simulink model "L3_T2_cascade_position"  (R2026a)
settings: Solver=ode23tb  StartTime=0  StopTime=4  MaxStep=0.001
settings Model: Creator=m  LastModifiedBy=m

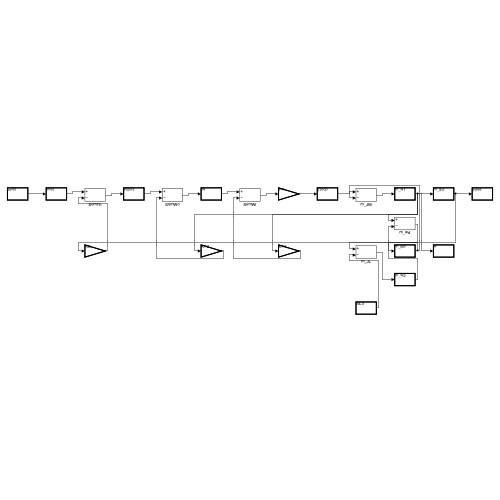
[thumbnail: Simulink's stored preview of the top-level diagram]
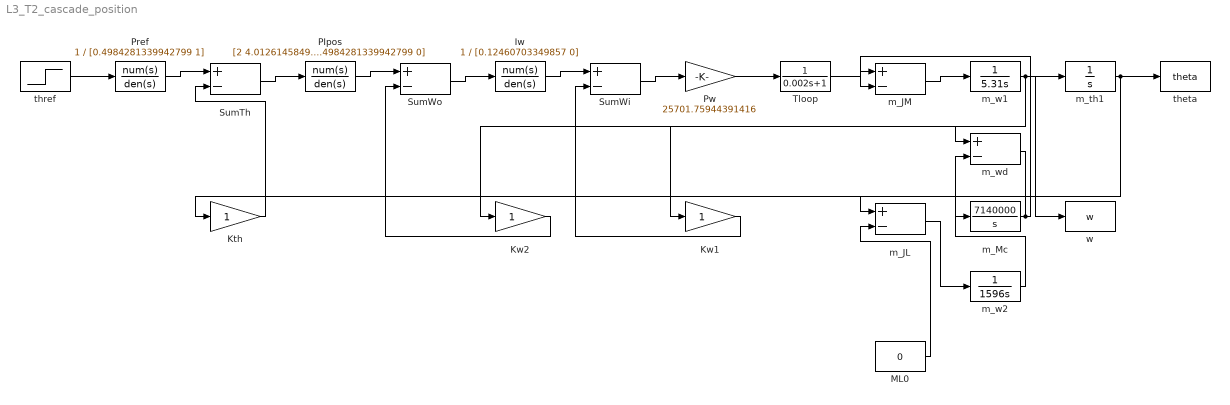
== system L3_T2_cascade_position ==
  Iw : TransferFcn  Numerator=1  Denominator=[0.12460703349857 0]
  Kth : Gain
  Kw1 : Gain
  Kw2 : Gain
  ML0 : Constant  Value=0
  PIpos : TransferFcn  Numerator=[2 4.012614584920185]  Denominator=[0.4984281339942799 0]
  Pref : TransferFcn  Numerator=1  Denominator=[0.4984281339942799 1]
  Pw : Gain  Gain=25701.75944391416
  SumTh : Sum  Inputs=+-
  SumWi : Sum  Inputs=+-
  SumWo : Sum  Inputs=+-
  Tloop : TransferFcn  Numerator=1  Denominator=[0.002 1]
  m_JL : Sum  Inputs=+-
  m_JM : Sum  Inputs=+-
  m_Mc : TransferFcn  Numerator=7140000  Denominator=[1 0]
  m_th1 : Integrator
  m_w1 : TransferFcn  Numerator=1  Denominator=[5.31 0]
  m_w2 : TransferFcn  Numerator=1  Denominator=[1596 0]
  m_wd : Sum  Inputs=+-
  theta : ToWorkspace  VariableName=theta  SaveFormat=Structure With Time  SampleTime=-1
  thref : Step  Time=0  FinalValue=0.08726646259971647  SampleTime=0
  w : ToWorkspace  VariableName=w  SaveFormat=Structure With Time  SampleTime=-1
  wires:
  m_JM/1 -> m_w1/1
  m_w1/1 -> m_wd/1, m_th1/1, Kw1/1, Kw2/1, w/1
  m_w2/1 -> m_wd/2
  m_wd/1 -> m_Mc/1
  m_Mc/1 -> m_JM/2, m_JL/1
  m_JL/1 -> m_w2/1
  thref/1 -> Pref/1
  Pref/1 -> SumTh/1
  SumTh/1 -> PIpos/1
  PIpos/1 -> SumWo/1
  SumWo/1 -> Iw/1
  Iw/1 -> SumWi/1
  SumWi/1 -> Pw/1
  Pw/1 -> Tloop/1
  Tloop/1 -> m_JM/1
  ML0/1 -> m_JL/2
  Kw1/1 -> SumWi/2
  Kw2/1 -> SumWo/2
  m_th1/1 -> Kth/1, theta/1
  Kth/1 -> SumTh/2
